simulink model "inputfilter"  (R2025b)
settings: Solver=VariableStepAuto  StartTime=0.0  StopTime=3  RelTol=1e-3
model workspace (MAT data in the model file):
  wn = 60
  xi = 1
undefined symbols (not defined in the file or in its folder): DiscIntNeverNeededParam
settings Model: Creator=yeqinghua  LastModifiedBy=yeqinghua

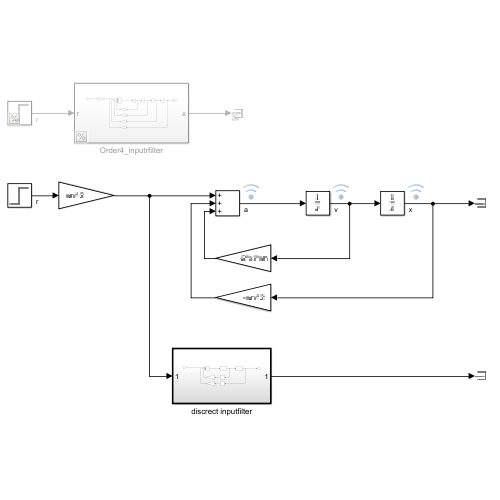
[thumbnail: Simulink's stored preview of the top-level diagram]
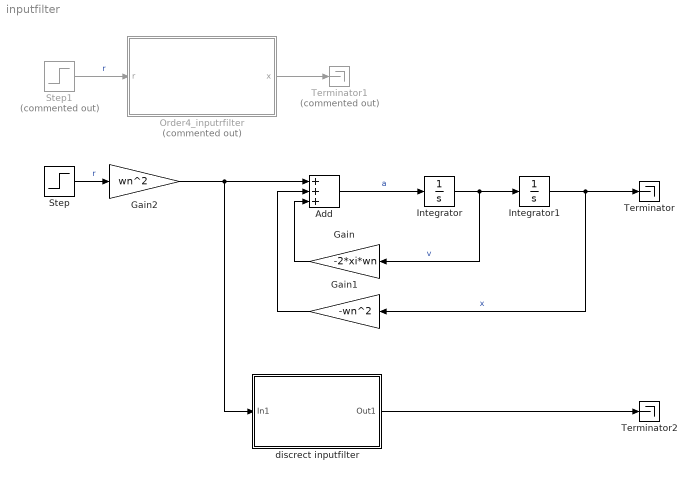
== system inputfilter ==
  Add : Sum  Inputs=+++
  Gain : Gain  Gain=-2*xi*wn
  Gain1 : Gain  Gain=-wn^2
  Gain2 : Gain  Gain=wn^2
  Integrator : Integrator
  Integrator1 : Integrator
  Order4_inputrfilter : Subsystem  Commented=on
  Step : Step  Time=0.001  After=0.002  SampleTime=0
  Step1 : Step  Commented=on  Time=0.001  After=0.02  SampleTime=0
  Terminator : Terminator
  Terminator1 : Terminator  Commented=on
  Terminator2 : Terminator
  discrect inputfilter : Subsystem  TreatAsAtomicUnit=on  SystemSampleTime=1e-6
  wires:
  Integrator/1 -> Gain/1, Integrator1/1  "v"
  Integrator1/1 -> Gain1/1, Terminator/1  "x"
  Add/1 -> Integrator/1  "a"
  Gain2/1 -> discrect inputfilter/1(In1), Add/1
  Gain/1 -> Add/3
  Gain1/1 -> Add/2
  Step/1 -> Gain2/1  "r"
  Step1/1 -> Order4_inputrfilter/1(r)  "r"
  Order4_inputrfilter/1(x) -> Terminator1/1
  discrect inputfilter/1(Out1) -> Terminator2/1

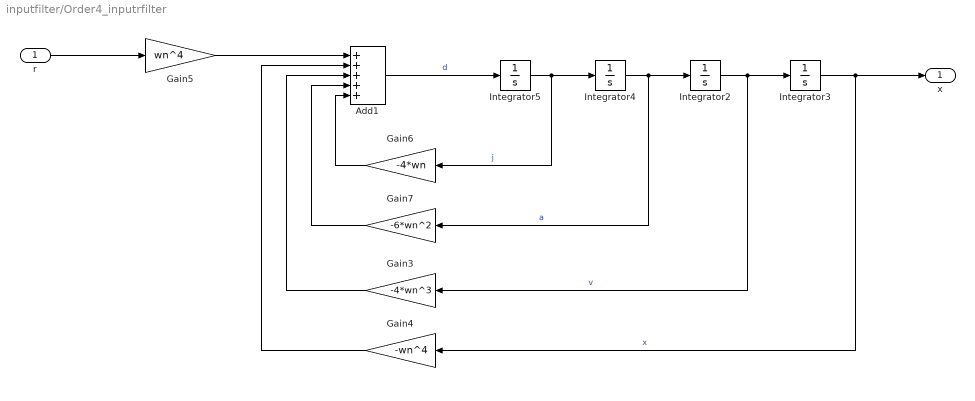
== system inputfilter/Order4_inputrfilter ==
  r : Inport
  Add1 : Sum  Inputs=+++++
  Gain3 : Gain  Gain=-4*wn^3
  Gain4 : Gain  Gain=-wn^4
  Gain5 : Gain  Gain=wn^4
  Gain6 : Gain  Gain=-4*wn
  Gain7 : Gain  Gain=-6*wn^2
  Integrator{2..5} (4 alike) : Integrator
  x : Outport
  wires:
  Add1/1 -> Integrator5/1  "d"
  Integrator4/1 -> Gain7/1, Integrator2/1  "a"
  Gain4/1 -> Add1/2
  Integrator5/1 -> Gain6/1, Integrator4/1  "j"
  Integrator3/1 -> x/1, Gain4/1  "x"
  Integrator2/1 -> Gain3/1, Integrator3/1  "v"
  Gain6/1 -> Add1/5
  Gain7/1 -> Add1/4
  Gain5/1 -> Add1/1
  Gain3/1 -> Add1/3
  r/1 -> Gain5/1

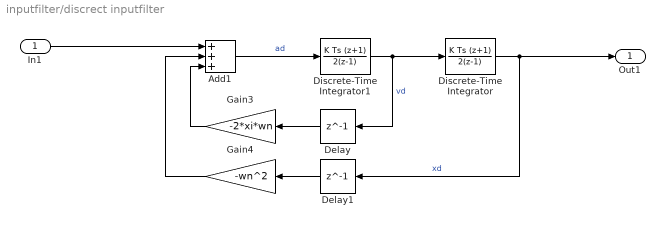
== system inputfilter/discrect inputfilter ==
  In1 : Inport
  Add1 : Sum  Inputs=+++
  Delay : Delay  DelayLength=1
  Delay1 : Delay  DelayLength=1
  Discrete-Time Integrator : DiscreteIntegrator  IntegratorMethod=Integration: Trapezoidal  SampleTime=-1  ICPrevOutput=DiscIntNeverNeededParam  ICPrevScaledInput=DiscIntNeverNeededParam
  Discrete-Time Integrator1 : DiscreteIntegrator  IntegratorMethod=Integration: Trapezoidal  SampleTime=-1  ICPrevOutput=DiscIntNeverNeededParam  ICPrevScaledInput=DiscIntNeverNeededParam
  Gain3 : Gain  Gain=-2*xi*wn
  Gain4 : Gain  Gain=-wn^2
  Out1 : Outport
  wires:
  In1/1 -> Add1/1
  Add1/1 -> Discrete-Time Integrator1/1  "ad"
  Gain3/1 -> Add1/3
  Discrete-Time Integrator/1 -> Out1/1, Delay1/1  "xd"
  Gain4/1 -> Add1/2
  Discrete-Time Integrator1/1 -> Delay/1, Discrete-Time Integrator/1  "vd"
  Delay/1 -> Gain3/1
  Delay1/1 -> Gain4/1
